simulink model "xianyu_jinji_steer_avoid_collision_add_y_and_alpha"  (R2021a)
settings: Solver=FixedStepAuto  StartTime=0.0  StopTime=6  FixedStep=0.001  RelTol=1e-3
PostLoadFcn:
  | , if any(exist('dsrtsu_mdlpostloadfcn', 'file') == [2, 3, 6]), try dsrtsu_mdlpostloadfcn('Execute', bdroot); catch fprintf('Error in PostLoadFcn (dsrtsu_mdlpostloadfcn) for model "%s":\n %s\n', bdroot, lasterr); end, end,
libraries: Solver_SF x1, simulink x1
settings Model: DSRTSU_INTERNAL_RTI_VER=500  DSRTSU_INTERNAL_RTI_TYPE=rti1401  DSRTSU_INTERNAL_RTIFPGA=90  Creator=11387  LastModifiedBy=yanglu
settings SolverCC: AlgebraicLoopSolver=TrustRegion
settings DataIOCC: ReturnWorkspaceOutputs=off
settings OptimizationCC: BlockReduction=off  OptimizeBlockIOStorage=off  BufferReuse=off  GlobalBufferReuse=off  ExpressionFolding=off  LocalBlockOutputs=off
settings DebuggingCC: SFMachineParentedDataDiag=warning  ArithmeticOperatorsInVariantConditions=warning
settings HardwareCC: ProdBitPerPointer=32  ProdBitPerSizeT=32  ProdBitPerPtrDiffT=32  ProdLargestAtomicInteger=Integer  ProdEndianess=BigEndian  ProdWordSize=32  ProdHWDeviceType=Custom Processor->Custom  TargetIntDivRoundTo=Zero  TargetEndianess=BigEndian  TargetHWDeviceType=Custom Processor->Custom
settings SFSimCC: SimUseLocalCustomCode=off  CustomCodeUndefinedFunction=UseInterfaceOnly
settings RTWCC: Description=dSPACE DS1401 Hardware Platform  SystemTargetFile=rti1401.tlc  MakeCommand=make_rti  TemplateMakefile=rti1401.tmf  RTWUseLocalCustomCode=off
settings CodeAppCC: StateflowObjectComments=on
settings STFCustomTargetCC: ParMdlRefBuildCompliant=on  MatFileLogging=on  GRTInterface=off  UseToolchainInfoCompliant=off  SystemTargetFile=rti1401.tlc
settings GRTTargetCC: TargetLangStandard=C89/C90 (ANSI)  CompOptLevelCompliant=off  ConcurrentExecutionCompliant=off  CombineOutputUpdateFcns=off  CPPClassGenCompliant=off  UseToolchainInfoCompliant=off
settings ConfigComp: CovMetricSettings=dswe

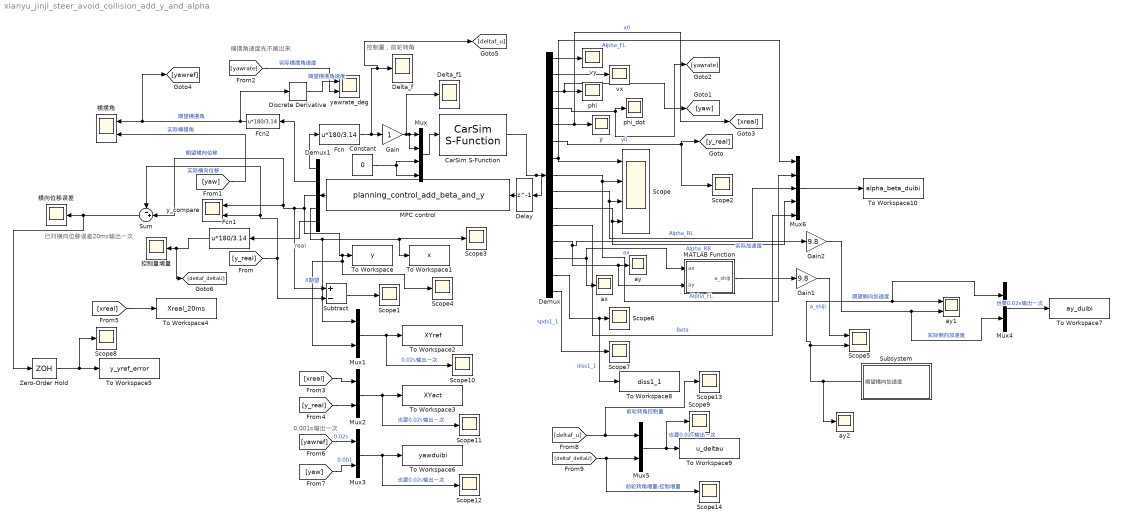
== system xianyu_jinji_steer_avoid_collision_add_y_and_alpha ==
  note: 0.001s输出一次
  note: 已对横向位移误差20ms输出一次
  note: 横摆角速度先不画出来
  note: 控制量，前轮转角
  note: real
  CarSim S-Function : Solver_SF/CarSim S-Function  Priority=1  SIMFILE=simfile.sim
  Constant : Constant  Value=0
  Delay : Delay  DelayLength=1  InitialCondition=0
  Delta_f : Scope
  Delta_f1 : Scope
  Demux : Demux  Outputs=15
  Demux1 : Demux  Outputs=5
  Discrete Derivative : simulink/Discrete/Discrete Derivative  gainval=1.0  ICPrevScaledInput=0.0  OutMin=[]  OutMax=[]  OutDataType=fixdt(1, 16)  OutScaling=2^-10  DoSatur=off
  Fcn : Fcn  Expr=u*180/3.14
  Fcn1 : Fcn  Expr=u*180/3.14
  Fcn2 : Fcn  Expr=u*180/3.14
  Gain : Gain
  Gain1 : Gain  Gain=9.8
  Gain2 : Gain  Gain=9.8
  MATLAB Function : MATLAB Function  TreatAsAtomicUnit=on
  MPC control : S-Function  FunctionName=planning_control_add_beta_and_y  SFunctionDeploymentMode=off  EnableBusSupport=off
  Mux : Mux
  Mux{1..5} (5 alike) : Mux  Inputs=2
  Mux6 : Mux  Inputs=5
  Scope : Scope  NumInputPorts=4
  Scope{1..4,6..14} (13 alike) : Scope
  Scope5 : Scope  NumInputPorts=2
  Subsystem : Subsystem
  Subtract : Sum  Inputs=+-
  Sum : Sum  Inputs=-+|
  To Workspace : ToWorkspace  VariableName=y  SampleTime=-1
  To Workspace1 : ToWorkspace  VariableName=x  SampleTime=-1
  To Workspace10 : ToWorkspace  VariableName=alpha_beta_duibi  SaveFormat=Timeseries  SampleTime=-1
      settings: Decimation=20
  To Workspace2 : ToWorkspace  VariableName=XYref  SaveFormat=Timeseries  SampleTime=-1
  To Workspace3 : ToWorkspace  VariableName=XYact  SaveFormat=Timeseries  SampleTime=-1
      settings: Decimation=20
  To Workspace4 : ToWorkspace  VariableName=Xreal_20ms  SaveFormat=Timeseries  SampleTime=-1
      settings: Decimation=20
  To Workspace5 : ToWorkspace  VariableName=y_yref_error  SaveFormat=Timeseries  SampleTime=-1
  To Workspace6 : ToWorkspace  VariableName=yawduibi  SaveFormat=Timeseries  SampleTime=-1
      settings: Decimation=20
  To Workspace7 : ToWorkspace  VariableName=ay_duibi  SaveFormat=Timeseries  SampleTime=-1
      settings: Decimation=20
  To Workspace8 : ToWorkspace  VariableName=diss1_1  SaveFormat=Timeseries  SampleTime=-1
      settings: Decimation=20
  To Workspace9 : ToWorkspace  VariableName=u_deltau  SaveFormat=Timeseries  SampleTime=-1
  Zero-Order Hold : ZeroOrderHold  SampleTime=0.02
  ax : Scope
  ay : Scope
  ay1 : Scope  NumInputPorts=2
  ay2 : Scope
  phi : Scope
  phi_dot : Scope
  vx : Scope
  vy : Scope
  y : Scope
  y_compare : Scope  NumInputPorts=2
  yawrate_deg : Scope  NumInputPorts=2
  控制量增量 : Scope
  横向位移误差 : Scope
  横摆角 : Scope  NumInputPorts=2
  wires:
  Fcn/1 -> [deltaf_u], Delta_f/1, Gain/1
  Delay/1 -> MPC control/1
  MPC control/1 -> Demux1/1
  Demux1/1 -> Fcn/1
  Demux/7 -> Scope/1, Mux6/1  "Alpha_FL"
  Demux/8 -> Mux6/2, Scope/2  "Alpha_FL"
  Demux/9 -> Mux6/3, Scope/3  "Alpha_RL"
  Demux/10 -> Mux6/4, Scope/4  "Alpha_RR"
  Demux/1 -> vy/1
  Demux/2 -> vx/1
  Demux/3 -> [yaw], phi/1
  Demux/4 -> [yawrate], phi_dot/1
  Demux/6 -> Scope2/1, [y_real]  "y0"
  Demux/11 -> Mux6/5  "Beta"
  Gain/1 -> Mux/2, Mux/1, Delta_f1/1
  Demux1/2 -> Fcn2/1
  Demux/5 -> [xreal], y/1  "x0"
  Subtract/1 -> Scope1/1
  Demux/12 -> MATLAB Function/2(ay), ay/1, Gain2/1  "实际加速度"
  CarSim S-Function/1 -> Delay/1, Demux/1
  Gain2/1 -> Mux4/2, ay1/2  "实际侧向加速度"
  Demux1/3 -> Mux1/2, Scope4/1, To Workspace/1, Subtract/1, Sum/2, y_compare/1  "期望横向位移"
  [y_real] -> Subtract/2, Sum/1, y_compare/2  "实际横向位移"
  [yaw] -> 横摆角/2  "实际横摆角"
  Fcn2/1 -> Discrete Derivative/1, [yawref], 横摆角/1  "期望横摆角"
  Subsystem/1(期望横向加速度) -> ay2/1, Mux4/1, ay1/1, Scope5/2  "期望侧向加速度"
  Demux1/4 -> Mux1/1, To Workspace1/1, Scope3/1  "X期望"
  Demux/13 -> ax/1, MATLAB Function/1(ax)  "ax"
  MATLAB Function/1(a_shiji) -> Gain1/1
  Gain1/1 -> Scope5/1  "a_shiji"
  Mux/1 -> CarSim S-Function/1
  Constant/1 -> Mux/3, Mux/4
  Demux1/5 -> Fcn1/1
  Fcn1/1 -> [deltaf_deltaU], 控制量增量/1
  [yawrate] -> yawrate_deg/2  "实际横摆角速度"
  Discrete Derivative/1 -> yawrate_deg/1  "期望横摆角速度"
  Demux/14 -> To Workspace8/1, Scope6/1  "diss1_1"
  Demux/15 -> Scope7/1  "spds1_1"
  Sum/1 -> Zero-Order Hold/1, 横向位移误差/1
  Mux1/1 -> Scope10/1, To Workspace2/1  "0.02s输出一次"
  [xreal] -> Mux2/1
  [y_real] -> Mux2/2
  Mux2/1 -> Scope11/1, To Workspace3/1  "也要0.02s输出一次"
  [xreal] -> To Workspace4/1
  Zero-Order Hold/1 -> Scope8/1, To Workspace5/1
  [yawref] -> Mux3/1  "0.02s"
  [yaw] -> Mux3/2  "0.001"
  Mux3/1 -> Scope12/1, To Workspace6/1  "也要0.02s输出一次"
  Mux4/1 -> To Workspace7/1  "也要0.02s输出一次"
  [deltaf_u] -> Scope13/1, Mux5/1  "前轮转角控制量"
  [deltaf_deltaU] -> Scope14/1, Mux5/2  "前轮转角增量/控制增量"
  Mux5/1 -> Scope9/1, To Workspace9/1  "也要0.02s输出一次"
  Mux6/1 -> To Workspace10/1

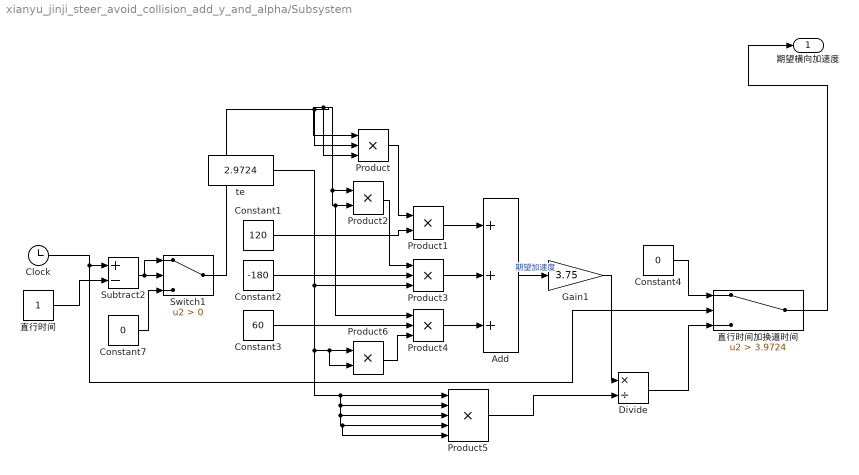
== system xianyu_jinji_steer_avoid_collision_add_y_and_alpha/Subsystem ==
  Add : Sum  Inputs=+++
  Clock : Clock
  Constant1 : Constant  Value=120
  Constant2 : Constant  Value=-180
  Constant3 : Constant  Value=60
  Constant4 : Constant  Value=0
  Constant7 : Constant  Value=0
  Divide : Product  Inputs=*/
  Gain1 : Gain  Gain=3.75
  Product : Product  Inputs=3
  Product1 : Product
  Product2 : Product
  Product3 : Product  Inputs=3
  Product4 : Product  Inputs=3
  Product5 : Product  Inputs=5
  Product6 : Product
  Subtract2 : Sum  Inputs=+-
  Switch1 : Switch  Criteria=u2 > Threshold
  te : Constant  Value=2.9724
  直行时间 : Constant
  直行时间加换道时间 : Switch  Criteria=u2 > Threshold  Threshold=3.9724
  期望横向加速度 : Outport
  wires:
  Clock/1 -> Subtract2/1, 直行时间加换道时间/2
  Product6/1 -> Product4/3
  直行时间加换道时间/1 -> 期望横向加速度/1
  Constant4/1 -> 直行时间加换道时间/1
  Divide/1 -> 直行时间加换道时间/3
  Constant3/1 -> Product4/2
  Constant2/1 -> Product3/2
  Subtract2/1 -> Switch1/1, Switch1/2
  Add/1 -> Gain1/1  "期望加速度"
  Constant1/1 -> Product1/2
  Product4/1 -> Add/3
  直行时间/1 -> Subtract2/2
  Product5/1 -> Divide/2
  Switch1/1 -> Product/1, Product4/1, Product2/2, Product2/1, Product/3, Product/2
  Constant7/1 -> Switch1/3
  Product2/1 -> Product3/1
  Product1/1 -> Add/1
  Product3/1 -> Add/2
  Product/1 -> Product1/1
  te/1 -> Product6/2, Product6/1, Product5/5, Product5/4, Product5/3, Product5/2, Product5/1, Product3/3
  Gain1/1 -> Divide/1

== matlab function xianyu_jinji_steer_avoid_collision_add_y_and_alpha/MATLAB Function ==
  data: ax input; a_shiji output; ay input
function a_shiji = fcn(ax,ay)
if ay>0
    a_shiji=sqrt(ax^2+ay^2);
else
    a_shiji=-sqrt(ax^2+ay^2);
end
